simulink model "ESP_sim"  (R2022b)
settings: Solver=VariableStepAuto  StartTime=0.0  StopTime=30  RelTol=1e-5
values from neighbouring files (symbols this model uses):
  vehicle_data = getVehicleDataStruct()    [main.m]
libraries: autolibshared x1
settings Model: Creator=ashkan  LastModifiedBy=ashkan

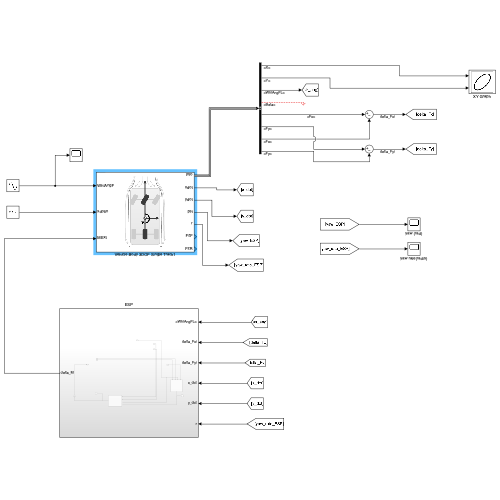
[thumbnail: Simulink's stored preview of the top-level diagram]
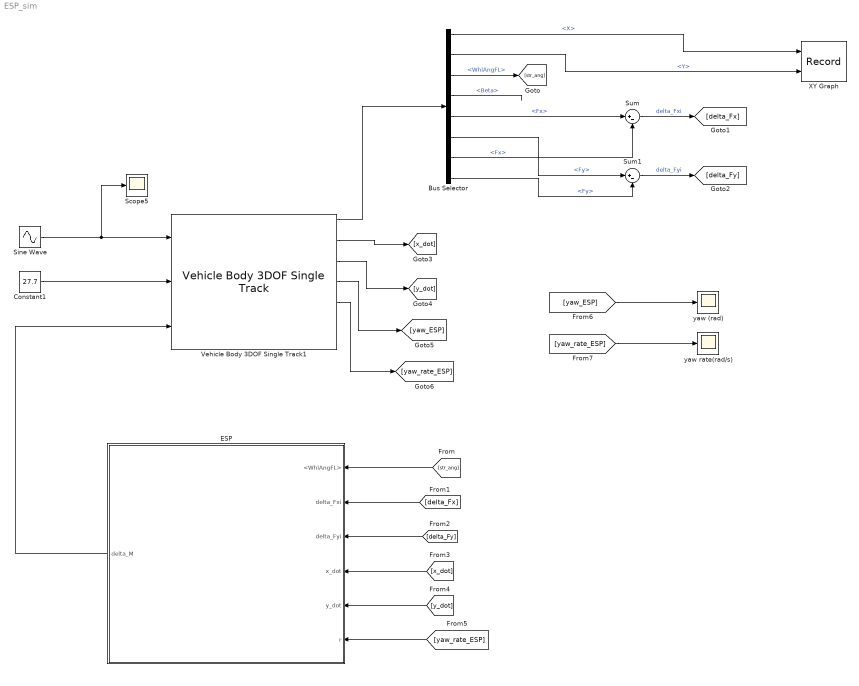
== system ESP_sim ==
  Bus Selector : BusSelector  OutputSignals=InertFrm.Cg.Disp.X,InertFrm.Cg.Disp.Y,BdyFrm.FrntAxl.Steer.WhlAngFL,BdyFrm.Cg.Ang.Beta,BdyFrm.Forces.RearAxl.Fx,BdyFrm.Forces.RearAxl.Fy,BdyFrm.Forces.FrntAxl.Fx,BdyFrm.Forces.FrntAxl.Fy
  Constant1 : Constant  Value=27.7
  ESP : Subsystem
  Scope5 : Scope
  Sine Wave : Sin  Amplitude=0.5  SampleTime=0
  Sum : Sum  Inputs=|+-
  Sum1 : Sum  Inputs=|+-
  Vehicle Body 3DOF Single Track1 : autolibshared/Vehicle Body 3DOF Single Track  trackMode=Single (bicycle)  inputMode=External longitudinal velocity  frontSteerMode=on  rearSteerMode=off  windMode=off  muMode=off  extFMode=off  extMMode=on  htchFMode=off  htchMMode=off  extXo=off  extpsio=off  extxdoto=off  extro=off  extYo=off  extTamb=off  extydoto=off  aMode=2  NF=2  NR=2  m=vehicle_data.vehicle.m  a=vehicle_data.vehicle.Lf  b=vehicle_data.vehicle.Lr  h=vehicle_data.vehicle.hGs  dh=1  hh=0.2  X_o=0  xdot_o=0  CalphaMode=off  sigmaMode=on  d=0  hl=0  w=[1.4,1.4]  Cy_f=vehicle_data.front_suspension.Ks_f  Cy_r=vehicle_data.rear_suspension.Ks_r  sigma_f=.1  sigma_r=.1  alpha_f_brk=[-.1 .1]  Cy_f_data=[-9e3 9e3]  alpha_r_brk=[-.1 .1]  Cy_r_data=[-9e3 9e3]  Y_o=0  ydot_o=0  Izz=vehicle_data.vehicle.i_zz  psi_o=0  r_o=0  Af=2  Cd=.3  Cl=.1  Cpm=.1  beta_w=[0 0.01:0.01:0.3]  Cs=[0 0.01:0.01:0.3]  Cym=[0 1e-6:0.01:0.3]  Pabs=101325  Tair=273  g=9.81  mu=1  xdot_tol=.01  Fznom=5000  Fxtire_sat=7e4  Fytire_sat=7e4  longOff=0  latOff=0  vertOff=0  wrapAng=off
  XY Graph : Record  FileSettingsInternal="{\"entries\":[{\"content\":{\"excelSettings\":{\"content\":{},\"type\":\"Streamout.ExcelSettings\"}},\"type\":\"Streamout.FileSettingStorage\",\"uuid\":\"26db1f1f-10a1-49e5-aa62-deb1133200b5\"}],\"packageUris\":[\"http://schema.mathworks.com/mf0/streamout_blocks/R2020a\"],\"version\":\"1.0\"}"  Layout=[1 1]  SignalsInternal="{\"entries\":[{\"content\":{\"signals\":[{\"content\":{\"blockPath\":[\"ESP_sim/XY Graph\"],\"channel\":[],\"dimensions\":[1],\"domain\":\"ESP_sim/XY Graph\",\"lineColor\":\"#a2142f\",\"plots\":[1],\"port\":1,\"sid\":[\"\"],\"signalID\":24530,\"signalName\":\"<X>\"},\"type\":\"RecordBlkView.Signal\",\"uuid\":\"0bf8b3e5-1dc3-469f-93de-2d924f9306da\"},{\"content\":{\"blockPath\":[\"ESP_sim/XY Graph\"],\"channel\":[],\"dimensions\":[1],\"domain\":\"ESP_sim/XY Graph\",\"lineColor\":\"#139fff\",\"plots\":[1],\"port\":2,\"sid\":[\"\"],\"signalID\":24534,\"signalName\":\"<Y>\"},\"type\":\"RecordBlkView.Signal\",\"uuid\":\"27a6b7a8-4096-4da8-b6f5-47dcdbb35058\"}]},\"type\":\"RecordBlkView.InputSignals\",\"uuid\":\"9b9c392b-e367-43eb-871a-5b477a32cc10\"}],\"packageUris\":[\"http://schema.mathworks.com/mf0/streamout_blocks/R2020a\"],\"version\":\"1.0\"}"  VisualizationBindings="{\"xyplotplugin\":{\"info\":[{\"series\":[{\"bindingParametersList\":[{\"parameter\":\"X-Axis\",\"signalID\":24530,\"signalName\":\"<X>\"},{\"parameter\":\"Y-Axis\",\"signalID\":24534,\"signalName\":\"<Y>\"}],\"seriesID\":6122}],\"subplotID\":1}]}}"  CompatibilityTag=XY
  yaw (rad) : Scope
  yaw rate(rad/s) : Scope
  wires:
  Bus Selector/4 -> ?  "<Beta>"
  Sum/1 -> [delta_Fx]  "delta_Fxi"
  [yaw_rate_ESP] -> ESP/6(r)
  Vehicle Body 3DOF Single Track1/5 -> [yaw_rate_ESP]
  [yaw_rate_ESP] -> yaw rate(rad/s)/1
  ESP/1(delta_M) -> Vehicle Body 3DOF Single Track1/3
  Constant1/1 -> Vehicle Body 3DOF Single Track1/2
  Bus Selector/2 -> XY Graph/2  "<Y>"
  [x_dot] -> ESP/4(x_dot)
  Bus Selector/1 -> XY Graph/1  "<X>"
  Vehicle Body 3DOF Single Track1/1 -> Bus Selector/1
  Bus Selector/5 -> Sum/1  "<Fx>"
  Bus Selector/8 -> Sum1/2  "<Fy>"
  Bus Selector/3 -> [str_ang]  "<WhlAngFL>"
  Bus Selector/6 -> Sum1/1  "<Fy>"
  Bus Selector/7 -> Sum/2  "<Fx>"
  [str_ang] -> ESP/1(<WhlAngFL>)
  [delta_Fx] -> ESP/2(delta_Fxi)
  Vehicle Body 3DOF Single Track1/4 -> [yaw_ESP]
  [delta_Fy] -> ESP/3(delta_Fyi)
  [yaw_ESP] -> yaw (rad)/1
  [y_dot] -> ESP/5(y_dot)
  Sine Wave/1 -> Scope5/1, Vehicle Body 3DOF Single Track1/1
  Vehicle Body 3DOF Single Track1/2 -> [x_dot]
  Vehicle Body 3DOF Single Track1/3 -> [y_dot]
  Sum1/1 -> [delta_Fy]  "delta_Fyi"

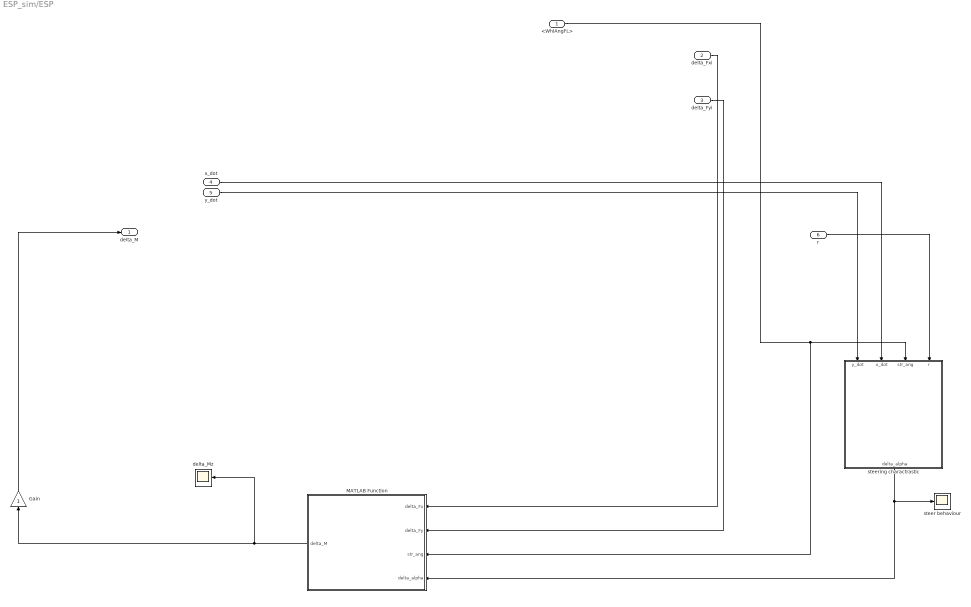
== system ESP_sim/ESP ==
  <WhlAngFL> : Inport
  delta_Fxi : Inport  Port=2
  delta_Fyi : Inport  Port=3
  x_dot : Inport  Port=4
  y_dot : Inport  Port=5
  r : Inport  Port=6
  Gain : Gain
  MATLAB Function : MATLAB Function  TreatAsAtomicUnit=on
  delta_Mz : Scope
  steer behaviour : Scope
  steering charactrastic : MATLAB Function  TreatAsAtomicUnit=on
  delta_M : Outport
  wires:
  x_dot/1 -> steering charactrastic/2(x_dot)
  delta_Fxi/1 -> MATLAB Function/1(delta_Fx)
  delta_Fyi/1 -> MATLAB Function/2(delta_Fy)
  steering charactrastic/1(delta_alpha) -> steer behaviour/1, MATLAB Function/4(delta_alpha)
  r/1 -> steering charactrastic/4(r)
  y_dot/1 -> steering charactrastic/1(y_dot)
  <WhlAngFL>/1 -> MATLAB Function/3(str_ang), steering charactrastic/3(str_ang)
  Gain/1 -> delta_M/1
  MATLAB Function/1(delta_M) -> Gain/1, delta_Mz/1

== matlab function ESP_sim/ESP/MATLAB Function ==
  data: delta_Fx input; delta_M output; delta_Fy input; str_ang input; delta_alpha input; vehicle_data parameter
function delta_M  = yaw_moment_diff(delta_Fx , delta_Fy ,  str_ang , delta_alpha , vehicle_data)

    a = vehicle_data.vehicle.Lf;
    b = vehicle_data.vehicle.Lr;
    L = vehicle_data.vehicle.L;

    if delta_alpha > 0      % over steering
        delta_Mz = (delta_Fx*(0.5*L*cos(str_ang) + a*sin(str_ang))) - (delta_Fy * (a*cos(str_ang) - 0.5*L*sin(str_ang)));


    elseif delta_alpha < 0  % under steering
        delta_Mz = (delta_Fx * 0.5*L) - (delta_Fy * b);


    else    % natural steering
        delta_Mz = 0;

    end

    delta_Mx = 0;
    delta_My = 0;

    delta_M = [delta_Mx , delta_My , delta_Mz];

end

== matlab function ESP_sim/ESP/steering charactrastic ==
  data: y_dot input; x_dot input; delta_alpha output; str_ang input; r input; vehicle_data parameter
function delta_alpha = steer_char(y_dot , x_dot , str_ang , r , vehicle_data)

    a = vehicle_data.vehicle.Lf;
    b = vehicle_data.vehicle.Lr;

    alpha_f = atan((y_dot + a*r)/(x_dot)) - str_ang;
    alpha_r = atan((y_dot - b*r)/(x_dot));

    delta_alpha = alpha_r - alpha_f;

end
